simulink model "Harvester_model"  (R2017a)
settings: Solver=FixedStepAuto  StartTime=0.0  StopTime=time(length(time))  FixedStep=1/fs  RelTol=1e-3
PreLoadFcn:
  | global m k b Z_l efficiency time current_data filtorder fc fs a_filtered displacement
values from neighbouring files (symbols this model uses):
  b = str2double(get(handles.b,'String'))    [Leg_motion_harvest_GUI.m]
  efficiency = (str2double(get(handles.efficiency,'String')))/100    [Leg_motion_harvest_GUI.m]
  k = ((2*pi*dom_freq)^2)*m    [Leg_motion_harvest_GUI.m]
  m = (str2double(get(handles.m,'String'))/1e3)    [Leg_motion_harvest_GUI.m]
  Z_l = (str2double(get(handles.Z_l,'String')))/1e3    [Leg_motion_harvest_GUI.m]
settings Model: Creator=mchi2cb3  LastModifiedBy=mchi2cb3

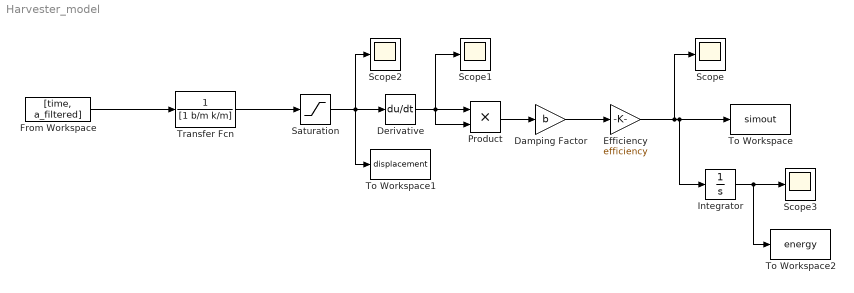
== system Harvester_model ==
  Damping Factor : Gain  Gain=b
  Derivative : Derivative
  Efficiency : Gain  Gain=efficiency
  From Workspace : FromWorkspace  VariableName=[time, a_filtered]  SampleTime=0
  Integrator : Integrator
  Product : Product
  Saturation : Saturate  UpperLimit=Z_l/2  LowerLimit=-Z_l/2
  Scope{,1..3} (4 alike) : Scope
  To Workspace : ToWorkspace  VariableName=simout  SaveFormat=Timeseries  SampleTime=-1
  To Workspace1 : ToWorkspace  VariableName=displacement  SaveFormat=Timeseries  SampleTime=-1
  To Workspace2 : ToWorkspace  VariableName=energy  SaveFormat=Timeseries  SampleTime=-1
  Transfer Fcn : TransferFcn  Denominator=[1 b/m k/m]
  wires:
  From Workspace/1 -> Transfer Fcn/1
  Transfer Fcn/1 -> Saturation/1
  Saturation/1 -> To Workspace1/1, Scope2/1, Derivative/1
  Product/1 -> Damping Factor/1
  Derivative/1 -> Scope1/1, Product/1, Product/2
  Damping Factor/1 -> Efficiency/1
  Efficiency/1 -> Integrator/1, To Workspace/1, Scope/1
  Integrator/1 -> To Workspace2/1, Scope3/1
